simulink model "FOC_Motor_Control"  (R2020b)
settings: Solver=FixedStepDiscrete  StartTime=0.0  StopTime=10.0  FixedStep=Fixed_Step_Size  RelTol=1e-3
values from neighbouring files (symbols this model uses):
  Angle = 1.0    [Hall_HFI_FOC_Data.sldd]
  Cosine_table = 1.0 0.99999529 0.99999058 0.99998587 0.99998116 0.99996704 0.99995291 0.99993885 0.99992472 0.99990118 0.99987763 0.99985409 0.9998306 0.99979764 0.99976468 0.99973178 0.99969882 0.99965644 0.99961412 0.99957174 0.99952942 0.99947762 0.99942589 0.99937415 0.99932235 0.9992612 0.99920005 0.99913889 0.99907768 0.99900717 0.99893659 0.99886602 0.99879545 0.99871546 0.99863547 0.99855554 0.99847555 0.    [Hall_HFI_FOC_Data.sldd]
  Flux = 0.00529276    [Hall_HFI_FOC_Data.sldd]
  HaLL_AngleShift = -0.25    [Hall_HFI_FOC_Data.sldd]
  HaLL_Sector1 = 5.236    [Hall_HFI_FOC_Data.sldd]
  HaLL_Sector2 = 1.0472    [Hall_HFI_FOC_Data.sldd]
  HaLL_Sector3 = 0.0    [Hall_HFI_FOC_Data.sldd]
  HaLL_Sector4 = 3.1415    [Hall_HFI_FOC_Data.sldd]
  HaLL_Sector5 = 4.1888    [Hall_HFI_FOC_Data.sldd]
  HaLL_Sector6 = 2.0944    [Hall_HFI_FOC_Data.sldd]
  HaLL_Timer_T = 1.0E-5    [Hall_HFI_FOC_Data.sldd]
  HFI_bw_BPF = 100.0    [Hall_HFI_FOC_Data.sldd]
  HFI_Fuc_Enalbe = 1.0    [Hall_HFI_FOC_Data.sldd]
  HFI_Inj_HF = 1000.0    [Hall_HFI_FOC_Data.sldd]
  HFI_Inj_HV = 2.0    [Hall_HFI_FOC_Data.sldd]
  HFI_IPD_F = 1000.0    [Hall_HFI_FOC_Data.sldd]
  HFI_IPD_Time = 0.1    [Hall_HFI_FOC_Data.sldd]
  HFI_IPD_V = 1.0    [Hall_HFI_FOC_Data.sldd]
  HFI_NS2RUN_Time = 0.1    [Hall_HFI_FOC_Data.sldd]
  HFI_NS_Low_Time = 0.01    [Hall_HFI_FOC_Data.sldd]
  HFI_NS_Time = 0.05    [Hall_HFI_FOC_Data.sldd]
  HFI_NS_V = 1.0    [Hall_HFI_FOC_Data.sldd]
  HFI_PLL_Omga = 50.0    [Hall_HFI_FOC_Data.sldd]
  HFI_PLL_Xi = 0.707    [Hall_HFI_FOC_Data.sldd]
  HFI_Pulse_Time = 0.001    [Hall_HFI_FOC_Data.sldd]
  HFI_Switch_Time = 0.1    [Hall_HFI_FOC_Data.sldd]
  ID_Ki = 45.0    [Hall_HFI_FOC_Data.sldd]
  ID_Kp = 0.4    [Hall_HFI_FOC_Data.sldd]
  IQ_Ki = 45.0    [Hall_HFI_FOC_Data.sldd]
  IQ_Kp = 0.45    [Hall_HFI_FOC_Data.sldd]
  LADRC_b0 = 80000.0    [Hall_HFI_FOC_Data.sldd]
  LADRC_Omega_c = 80.0    [Hall_HFI_FOC_Data.sldd]
  Ld = 0.0004    [Hall_HFI_FOC_Data.sldd]
  Lq = 0.00045    [Hall_HFI_FOC_Data.sldd]
  Over_modulation = 0.0    [Hall_HFI_FOC_Data.sldd]
  Pole_Pairs = 2.0    [Hall_HFI_FOC_Data.sldd]
  PWM_Frequency = 10000.0    [Hall_HFI_FOC_Data.sldd]
  Sine_table = 0.0 0.0015339879 0.0030679768 0.0046019657 0.0061359555 0.0076698866 0.0092038177 0.010737749 0.012271681 0.013805497 0.015339312 0.016873131 0.018406944 0.019940587 0.021474229 0.023007872 0.024541514 0.026074925 0.027608337 0.029141748 0.03067516 0.032208283 0.033741407 0.035274528 0.036807653 0.038340431 0.039873205 0.04140598 0.042938754 0.04447113 0.046003502 0.047535874 0.049068246 0.0506001    [Hall_HFI_FOC_Data.sldd]
  SMO_PLL_W = 50.0    [Hall_HFI_FOC_Data.sldd]
  Speed_Ki = 0.0633    [Hall_HFI_FOC_Data.sldd]
  Speed_Kp = 0.00867    [Hall_HFI_FOC_Data.sldd]
  Speed_PI_OutputMax = 6.0    [Hall_HFI_FOC_Data.sldd]
  Speed_PI_OutputMin = -6.0    [Hall_HFI_FOC_Data.sldd]
  SpeedFilter_Fn = 0.3    [Hall_HFI_FOC_Data.sldd]
  TorqueMode = 1.0    [Hall_HFI_FOC_Data.sldd]
undefined symbols (not defined in the file or in its folder): DiscIntNeverNeededParam, inverter, magnitude, SVPWM
libraries: simulink x6, eeGeneralControl x3, dspstat3 x3, pid_lib x1
(part 4 of 4)

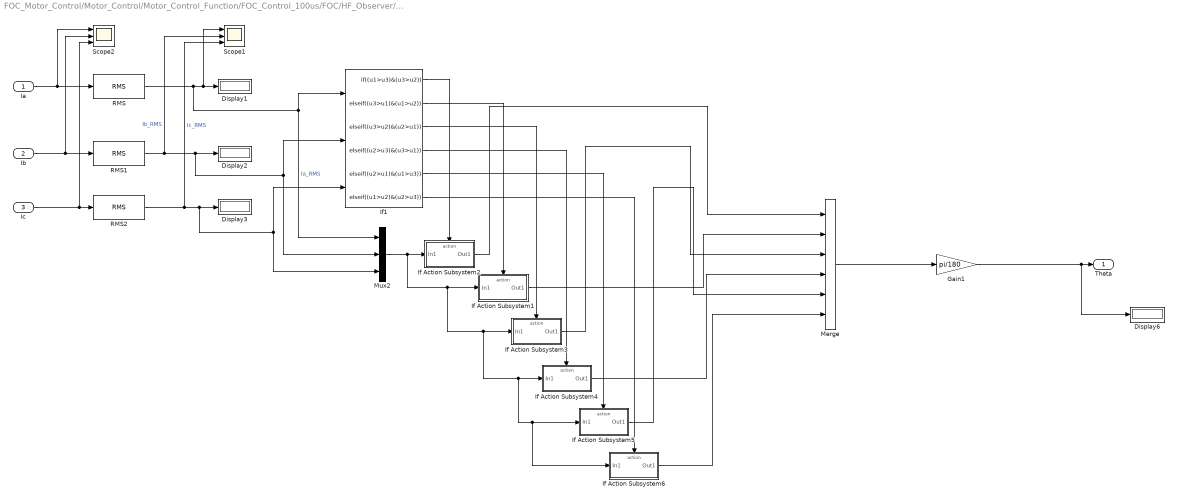
== system FOC_Motor_Control/Motor_Control/Motor_Control_Function/FOC_Control_100us/FOC/HF_Observer/HFI_Function/IPD/Theta_cacl ==
  Ia : Inport
  Ib : Inport  Port=2
  Ic : Inport  Port=3
  Display{1..3,6} (4 alike) : Display
  Gain1 : Gain  Gain=pi/180
  If Action Subsystem1 : Subsystem  TreatAsAtomicUnit=on
  If Action Subsystem2 : Subsystem  TreatAsAtomicUnit=on
  If Action Subsystem3 : Subsystem  TreatAsAtomicUnit=on
  If Action Subsystem4 : Subsystem  TreatAsAtomicUnit=on
  If Action Subsystem5 : Subsystem  TreatAsAtomicUnit=on
  If Action Subsystem6 : Subsystem  TreatAsAtomicUnit=on
  If1 : If  NumInputs=3  IfExpression=(u1>u3)&(u3>u2)  ElseIfExpressions=(u3>u1)&(u1>u2),(u3>u2)&(u2>u1),(u2>u3)&(u3>u1),(u2>u1)&(u1>u3),(u1>u2)&(u2>u3)  ShowElse=off
  Merge : Merge  Inputs=6
  Mux2 : Mux  Inputs=3
  RMS : dspstat3/RMS  run=on  directionMode=Each column  dimension=1  reset_popup=None
  RMS1 : dspstat3/RMS  run=on  directionMode=Each column  dimension=1  reset_popup=None
  RMS2 : dspstat3/RMS  run=on  directionMode=Each column  dimension=1  InputProcessing=Columns as channels (frame based)  reset_popup=None
  Scope1 : Scope  NumInputPorts=3
  Scope2 : Scope  NumInputPorts=3
  Theta : Outport
  wires:
  Ia/1 -> Scope2/1, RMS/1
  Ib/1 -> Scope2/2, RMS1/1
  Ic/1 -> Scope2/3, RMS2/1
  RMS2/1 -> If1/3, Mux2/3, Display3/1, Scope1/3  "Ic_RMS"
  RMS1/1 -> If1/2, Mux2/2, Display2/1, Scope1/2  "Ib_RMS"
  RMS/1 -> If1/1, Mux2/1, Display1/1, Scope1/1  "Ia_RMS"
  If1/1 -> If Action Subsystem2/Action
  If1/2 -> If Action Subsystem1/Action
  If1/3 -> If Action Subsystem3/Action
  If1/4 -> If Action Subsystem4/Action
  If1/5 -> If Action Subsystem5/Action
  If1/6 -> If Action Subsystem6/Action
  Mux2/1 -> If Action Subsystem6/1(In1), If Action Subsystem5/1(In1), If Action Subsystem4/1(In1), If Action Subsystem3/1(In1), If Action Subsystem1/1(In1), If Action Subsystem2/1(In1)
  If Action Subsystem2/1(Out1) -> Merge/1
  If Action Subsystem1/1(Out1) -> Merge/2
  If Action Subsystem3/1(Out1) -> Merge/3
  If Action Subsystem4/1(Out1) -> Merge/4
  If Action Subsystem5/1(Out1) -> Merge/5
  If Action Subsystem6/1(Out1) -> Merge/6
  Merge/1 -> Gain1/1
  Gain1/1 -> Display6/1, Theta/1

== system FOC_Motor_Control/Motor_Control/Motor_Control_Function/FOC_Control_100us/FOC/HF_Observer/HFI_Function/NS/Ud_inject_1 ==
  Theta : Inport
  Action Port : ActionPort  ActionPortLabel=case [ 1 ]:
  1 : Fcn  Expr=u[1]*u[4]-u[2]*u[3]
  2 : Fcn  Expr=u[1]*u[3]+u[2]*u[4]
  Constant : Constant  Value=0  OutDataTypeStr=single
  Constant2 : Constant  Value=0  OutDataTypeStr=single
  Mux : Mux
  Sine_Cosine : Subsystem  TreatAsAtomicUnit=on
      settings: RTWSystemCode=Nonreusable function  RTWFcnNameOpts=Use subsystem name
  Ualpha : Outport
  Ubeta : Outport  Port=2
  wires:
  Constant2/1 -> Mux/2
  Theta/1 -> Sine_Cosine/1(P)
  2/1 -> Ubeta/1
  Sine_Cosine/2(Cos) -> Mux/4
  1/1 -> Ualpha/1
  Constant/1 -> Mux/1
  Mux/1 -> 2/1, 1/1
  Sine_Cosine/1(Sin) -> Mux/3

== system FOC_Motor_Control/Motor_Control/Motor_Control_Function/FOC_Control_100us/FOC/HF_Observer/HFI_Function/NS/Ud_inject_2 ==
  Id : Inport
  Theta : Inport  Port=2
  Action Port : ActionPort  ActionPortLabel=case [ 2 ]:
  1 : Fcn  Expr=u[1]*u[4]-u[2]*u[3]
  2 : Fcn  Expr=u[1]*u[3]+u[2]*u[4]
  Constant : Constant  Value=HFI_NS_V  OutDataTypeStr=single
  Constant2 : Constant  Value=0  OutDataTypeStr=single
  Mux : Mux
  Sine_Cosine : Subsystem  TreatAsAtomicUnit=on
      settings: RTWSystemCode=Nonreusable function  RTWFcnNameOpts=Use subsystem name
  Ualpha : Outport
  Ubeta : Outport  Port=2
  Id_out : Outport  Port=3
  wires:
  Constant2/1 -> Mux/2
  Theta/1 -> Sine_Cosine/1(P)
  2/1 -> Ubeta/1
  Sine_Cosine/2(Cos) -> Mux/4
  1/1 -> Ualpha/1
  Constant/1 -> Mux/1
  Mux/1 -> 2/1, 1/1
  Sine_Cosine/1(Sin) -> Mux/3
  Id/1 -> Id_out/1

== system FOC_Motor_Control/Motor_Control/Motor_Control_Function/FOC_Control_100us/FOC/HF_Observer/HFI_Function/NS/Ud_inject_3 ==
  Theta : Inport
  Action Port : ActionPort  ActionPortLabel=case [ 3 ]:
  1 : Fcn  Expr=u[1]*u[4]-u[2]*u[3]
  2 : Fcn  Expr=u[1]*u[3]+u[2]*u[4]
  Constant : Constant  Value=0  OutDataTypeStr=single
  Constant2 : Constant  Value=0  OutDataTypeStr=single
  Mux : Mux
  Sine_Cosine : Subsystem  TreatAsAtomicUnit=on
      settings: RTWSystemCode=Nonreusable function  RTWFcnNameOpts=Use subsystem name
  Ualpha : Outport
  Ubeta : Outport  Port=2
  wires:
  Constant2/1 -> Mux/2
  Theta/1 -> Sine_Cosine/1(P)
  2/1 -> Ubeta/1
  Sine_Cosine/2(Cos) -> Mux/4
  1/1 -> Ualpha/1
  Constant/1 -> Mux/1
  Mux/1 -> 2/1, 1/1
  Sine_Cosine/1(Sin) -> Mux/3

== system FOC_Motor_Control/Motor_Control/Motor_Control_Function/FOC_Control_100us/FOC/HF_Observer/HFI_Function/NS/Ud_inject_4 ==
  Id : Inport
  Theta : Inport  Port=2
  Action Port : ActionPort  ActionPortLabel=case [ 4 ]:
  1 : Fcn  Expr=u[1]*u[4]-u[2]*u[3]
  2 : Fcn  Expr=u[1]*u[3]+u[2]*u[4]
  Constant : Constant  Value=HFI_NS_V  OutDataTypeStr=single
  Constant2 : Constant  Value=0  OutDataTypeStr=single
  Mux : Mux
  Sine_Cosine : Subsystem  TreatAsAtomicUnit=on
      settings: RTWSystemCode=Nonreusable function
  Theta_limit : Subsystem
      settings: RTWSystemCode=Nonreusable function
  Ualpha : Outport
  Ubeta : Outport  Port=2
  Id_out : Outport  Port=3
  wires:
  Constant2/1 -> Mux/2
  2/1 -> Ubeta/1
  Sine_Cosine/2(Cos) -> Mux/4
  1/1 -> Ualpha/1
  Constant/1 -> Mux/1
  Mux/1 -> 2/1, 1/1
  Sine_Cosine/1(Sin) -> Mux/3
  Id/1 -> Id_out/1
  Theta_limit/1(Angle_output) -> Sine_Cosine/1(P)
  Theta/1 -> Theta_limit/1(Angle_input)

== system FOC_Motor_Control/Motor_Control/Motor_Control_Function/FOC_Control_100us/FOC/HF_Observer/HFI_Function/NS/Ud_inject_5 ==
  Theta : Inport
  Id1 : Inport  Port=2
  Id2 : Inport  Port=3
  Action Port : ActionPort  ActionPortLabel=case [ 5 ]:
  1 : Fcn  Expr=u[1]*u[4]-u[2]*u[3]
  2 : Fcn  Expr=u[1]*u[3]+u[2]*u[4]
  Constant : Constant  Value=0  OutDataTypeStr=single
  Constant2 : Constant  Value=0  OutDataTypeStr=single
  If1 : If  NumInputs=2  IfExpression=u1>=u2  ElseIfExpressions=u1<u2  ShowElse=off
  Merge1 : Merge
  Mux : Mux
  Sine_Cosine : Subsystem
      settings: RTWSystemCode=Nonreusable function  RTWFcnNameOpts=Use subsystem name
  Subsystem : Subsystem
  Subsystem1 : Subsystem
  Ualpha : Outport
  Ubeta : Outport  Port=2
  IPD_Angle : Outport  Port=3
  wires:
  Constant2/1 -> Mux/2
  Theta/1 -> Subsystem1/1(In1), Subsystem/1(In1), Sine_Cosine/1(P)
  2/1 -> Ubeta/1
  Sine_Cosine/2(Cos) -> Mux/4
  1/1 -> Ualpha/1
  Constant/1 -> Mux/1
  Mux/1 -> 2/1, 1/1
  Sine_Cosine/1(Sin) -> Mux/3
  Id1/1 -> If1/1
  Id2/1 -> If1/2
  If1/1 -> Subsystem/Action
  If1/2 -> Subsystem1/Action
  Subsystem/1(Out1) -> Merge1/1
  Subsystem1/1(Out1) -> Merge1/2
  Merge1/1 -> IPD_Angle/1

== system FOC_Motor_Control/Motor_Control/Motor_Control_Function/FOC_Control_100us/FOC/HF_Observer/HFI_Function/HFI/IPD_Angle/Angle_calibration ==
  Angle_input : Inport
  Angle_offset : Constant  Value=-pi  OutDataTypeStr=single
  If Action Subsystem1 : Subsystem  TreatAsAtomicUnit=on
  If Action Subsystem2 : Subsystem  TreatAsAtomicUnit=on
  If Action Subsystem3 : Subsystem  TreatAsAtomicUnit=on
  If1 : If  IfExpression=u1 > 6.283185307  ElseIfExpressions=u1<0
  Merge1 : Merge  Inputs=3
  Subtract1 : Sum
  Angle_output : Outport
  wires:
  Angle_input/1 -> Subtract1/1
  Angle_offset/1 -> Subtract1/2  "Control_ModeCommand"
  If1/1 -> If Action Subsystem2/Action
  If1/3 -> If Action Subsystem1/Action
  If Action Subsystem2/1(Out1) -> Merge1/1
  Subtract1/1 -> If Action Subsystem3/1(In1), If Action Subsystem1/1(In1), If Action Subsystem2/1(In1), If1/1
  If Action Subsystem1/1(Out1) -> Merge1/3
  If Action Subsystem3/1(Out1) -> Merge1/2
  If1/2 -> If Action Subsystem3/Action
  Merge1/1 -> Angle_output/1

== system FOC_Motor_Control/Motor_Control/Motor_Control_Function/FOC_Control_100us/FOC/HF_Observer/HFI_Function/HFI/IPD_Angle1/Angle_calibration ==
  Angle_input : Inport
  Angle_offset : Constant  Value=pi  OutDataTypeStr=single
  If Action Subsystem1 : Subsystem  TreatAsAtomicUnit=on
  If Action Subsystem2 : Subsystem  TreatAsAtomicUnit=on
  If Action Subsystem3 : Subsystem  TreatAsAtomicUnit=on
  If1 : If  IfExpression=u1 > 6.283185307  ElseIfExpressions=u1<0
  Merge1 : Merge  Inputs=3
  Subtract1 : Sum
  Angle_output : Outport
  wires:
  Angle_input/1 -> Subtract1/1
  Angle_offset/1 -> Subtract1/2  "Control_ModeCommand"
  If1/1 -> If Action Subsystem2/Action
  If1/3 -> If Action Subsystem1/Action
  If Action Subsystem2/1(Out1) -> Merge1/1
  Subtract1/1 -> If Action Subsystem3/1(In1), If Action Subsystem1/1(In1), If Action Subsystem2/1(In1), If1/1
  If Action Subsystem1/1(Out1) -> Merge1/3
  If Action Subsystem3/1(Out1) -> Merge1/2
  If1/2 -> If Action Subsystem3/Action
  Merge1/1 -> Angle_output/1

== system FOC_Motor_Control/Motor_Control/Motor_Control_Function/FOC_Control_100us/FOC/HF_Observer/HFI_Function/HFI/Subsystem/Sine_Cosine ==
  note: Sine Cosine Coefficients
  P : Inport
  Cosine : Lookup_n-D  NumberOfTableDimensions=1  LookupTableObject=''  BreakpointsForDimension1=[0:2*pi/4095:2*pi]  BreakpointsForDimension1FirstPoint=10  BreakpointsForDimension2FirstPoint=10  BreakpointsForDimension1Spacing=12  BreakpointsForDimension2Spacing=12  IndexSearchMethod=Evenly spaced points  Table=Cosine_table  InterpMethod=Flat  DiagnosticForOutOfRangeInput=Error  InternalRulePriority=Speed  RndMeth=Simplest  InputSameDT=on
  Saturation : Saturate  UpperLimit=2*pi-0.001  LowerLimit=0+0.001
  Scope : Scope  NumInputPorts=2
  Sine : Lookup_n-D  NumberOfTableDimensions=1  LookupTableObject=''  BreakpointsForDimension1=[0:2*pi/4095:2*pi]  BreakpointsForDimension1FirstPoint=10  BreakpointsForDimension2FirstPoint=10  BreakpointsForDimension1Spacing=12  BreakpointsForDimension2Spacing=12  IndexSearchMethod=Evenly spaced points  Table=Sine_table  InterpMethod=Flat  DiagnosticForOutOfRangeInput=Error  InternalRulePriority=Speed  RndMeth=Simplest  InputSameDT=on
  Sin : Outport  VectorParamsAs1DForOutWhenUnconnected=off
  Cos : Outport  Port=2  VectorParamsAs1DForOutWhenUnconnected=off
  wires:
  P/1 -> Saturation/1  "position"
  Sine/1 -> Scope/1, Sin/1
  Cosine/1 -> Scope/2, Cos/1
  Saturation/1 -> Cosine/1, Sine/1

== system FOC_Motor_Control/Motor_Control/Motor_Control_Function/FOC_Control_100us/FOC/HF_Observer/HFI_Function/IPD/Theta_cacl/If Action Subsystem1 ==
  In1 : Inport
  Action Port : ActionPort  ActionPortLabel=elseif((u3>u1)&(u1>u2))
  Fcn : Fcn  Expr=(u(3)-u(1))/(u(3)-u(2))*30+30
  Out1 : Outport
  wires:
  In1/1 -> Fcn/1
  Fcn/1 -> Out1/1

== system FOC_Motor_Control/Motor_Control/Motor_Control_Function/FOC_Control_100us/FOC/HF_Observer/HFI_Function/IPD/Theta_cacl/If Action Subsystem2 ==
  In1 : Inport
  Action Port : ActionPort  ActionPortLabel=if((u1>u3)&(u3>u2))
  Fcn : Fcn  Expr=(u(3)-u(2))/(u(1)-u(2))*30
  Out1 : Outport
  wires:
  In1/1 -> Fcn/1
  Fcn/1 -> Out1/1

== system FOC_Motor_Control/Motor_Control/Motor_Control_Function/FOC_Control_100us/FOC/HF_Observer/HFI_Function/IPD/Theta_cacl/If Action Subsystem3 ==
  In1 : Inport
  Action Port : ActionPort  ActionPortLabel=elseif((u3>u2)&(u2>u1))
  Fcn : Fcn  Expr=(u(2)-u(1))/(u(3)-u(1))*30+60
  Out1 : Outport
  wires:
  In1/1 -> Fcn/1
  Fcn/1 -> Out1/1

== system FOC_Motor_Control/Motor_Control/Motor_Control_Function/FOC_Control_100us/FOC/HF_Observer/HFI_Function/IPD/Theta_cacl/If Action Subsystem4 ==
  In1 : Inport
  Action Port : ActionPort  ActionPortLabel=elseif((u2>u3)&(u3>u1))
  Fcn : Fcn  Expr=(u(2)-u(3))/(u(2)-u(1))*30+90
  Out1 : Outport
  wires:
  In1/1 -> Fcn/1
  Fcn/1 -> Out1/1

== system FOC_Motor_Control/Motor_Control/Motor_Control_Function/FOC_Control_100us/FOC/HF_Observer/HFI_Function/IPD/Theta_cacl/If Action Subsystem5 ==
  In1 : Inport
  Action Port : ActionPort  ActionPortLabel=elseif((u2>u1)&(u1>u3))
  Fcn : Fcn  Expr=(u(1)-u(3))/(u(2)-u(3))*30+120
  Out1 : Outport
  wires:
  In1/1 -> Fcn/1
  Fcn/1 -> Out1/1

== system FOC_Motor_Control/Motor_Control/Motor_Control_Function/FOC_Control_100us/FOC/HF_Observer/HFI_Function/IPD/Theta_cacl/If Action Subsystem6 ==
  In1 : Inport
  Action Port : ActionPort  ActionPortLabel=elseif((u1>u2)&(u2>u3))
  Fcn : Fcn  Expr=(u(1)-u(2))/(u(1)-u(3))*30+150
  Out1 : Outport
  wires:
  In1/1 -> Fcn/1
  Fcn/1 -> Out1/1

== system FOC_Motor_Control/Motor_Control/Motor_Control_Function/FOC_Control_100us/FOC/HF_Observer/HFI_Function/NS/Ud_inject_1/Sine_Cosine ==
  note: Sine Cosine Coefficients
  P : Inport
  Cosine : Lookup_n-D  NumberOfTableDimensions=1  LookupTableObject=''  BreakpointsForDimension1=[0:2*pi/4095:2*pi]  BreakpointsForDimension1FirstPoint=10  BreakpointsForDimension2FirstPoint=10  BreakpointsForDimension1Spacing=12  BreakpointsForDimension2Spacing=12  IndexSearchMethod=Evenly spaced points  Table=Cosine_table  InterpMethod=Flat  DiagnosticForOutOfRangeInput=Error  InternalRulePriority=Speed  RndMeth=Simplest  InputSameDT=on
  Scope : Scope  NumInputPorts=2
  Sine : Lookup_n-D  NumberOfTableDimensions=1  LookupTableObject=''  BreakpointsForDimension1=[0:2*pi/4095:2*pi]  BreakpointsForDimension1FirstPoint=10  BreakpointsForDimension2FirstPoint=10  BreakpointsForDimension1Spacing=12  BreakpointsForDimension2Spacing=12  IndexSearchMethod=Evenly spaced points  Table=Sine_table  InterpMethod=Flat  DiagnosticForOutOfRangeInput=Error  InternalRulePriority=Speed  RndMeth=Simplest  InputSameDT=on
  Sin : Outport  VectorParamsAs1DForOutWhenUnconnected=off
  Cos : Outport  Port=2  VectorParamsAs1DForOutWhenUnconnected=off
  wires:
  P/1 -> Cosine/1, Sine/1  "position"
  Sine/1 -> Scope/1, Sin/1
  Cosine/1 -> Scope/2, Cos/1

== system FOC_Motor_Control/Motor_Control/Motor_Control_Function/FOC_Control_100us/FOC/HF_Observer/HFI_Function/NS/Ud_inject_2/Sine_Cosine ==
  note: Sine Cosine Coefficients
  P : Inport
  Cosine : Lookup_n-D  NumberOfTableDimensions=1  LookupTableObject=''  BreakpointsForDimension1=[0:2*pi/4095:2*pi]  BreakpointsForDimension1FirstPoint=10  BreakpointsForDimension2FirstPoint=10  BreakpointsForDimension1Spacing=12  BreakpointsForDimension2Spacing=12  IndexSearchMethod=Evenly spaced points  Table=Cosine_table  InterpMethod=Flat  DiagnosticForOutOfRangeInput=Error  InternalRulePriority=Speed  RndMeth=Simplest  InputSameDT=on
  Scope : Scope  NumInputPorts=2
  Sine : Lookup_n-D  NumberOfTableDimensions=1  LookupTableObject=''  BreakpointsForDimension1=[0:2*pi/4095:2*pi]  BreakpointsForDimension1FirstPoint=10  BreakpointsForDimension2FirstPoint=10  BreakpointsForDimension1Spacing=12  BreakpointsForDimension2Spacing=12  IndexSearchMethod=Evenly spaced points  Table=Sine_table  InterpMethod=Flat  DiagnosticForOutOfRangeInput=Error  InternalRulePriority=Speed  RndMeth=Simplest  InputSameDT=on
  Sin : Outport  VectorParamsAs1DForOutWhenUnconnected=off
  Cos : Outport  Port=2  VectorParamsAs1DForOutWhenUnconnected=off
  wires:
  P/1 -> Cosine/1, Sine/1  "position"
  Sine/1 -> Scope/1, Sin/1
  Cosine/1 -> Scope/2, Cos/1

== system FOC_Motor_Control/Motor_Control/Motor_Control_Function/FOC_Control_100us/FOC/HF_Observer/HFI_Function/NS/Ud_inject_3/Sine_Cosine ==
  note: Sine Cosine Coefficients
  P : Inport
  Cosine : Lookup_n-D  NumberOfTableDimensions=1  LookupTableObject=''  BreakpointsForDimension1=[0:2*pi/4095:2*pi]  BreakpointsForDimension1FirstPoint=10  BreakpointsForDimension2FirstPoint=10  BreakpointsForDimension1Spacing=12  BreakpointsForDimension2Spacing=12  IndexSearchMethod=Evenly spaced points  Table=Cosine_table  InterpMethod=Flat  DiagnosticForOutOfRangeInput=Error  InternalRulePriority=Speed  RndMeth=Simplest  InputSameDT=on
  Scope : Scope  NumInputPorts=2
  Sine : Lookup_n-D  NumberOfTableDimensions=1  LookupTableObject=''  BreakpointsForDimension1=[0:2*pi/4095:2*pi]  BreakpointsForDimension1FirstPoint=10  BreakpointsForDimension2FirstPoint=10  BreakpointsForDimension1Spacing=12  BreakpointsForDimension2Spacing=12  IndexSearchMethod=Evenly spaced points  Table=Sine_table  InterpMethod=Flat  DiagnosticForOutOfRangeInput=Error  InternalRulePriority=Speed  RndMeth=Simplest  InputSameDT=on
  Sin : Outport  VectorParamsAs1DForOutWhenUnconnected=off
  Cos : Outport  Port=2  VectorParamsAs1DForOutWhenUnconnected=off
  wires:
  P/1 -> Cosine/1, Sine/1  "position"
  Sine/1 -> Scope/1, Sin/1
  Cosine/1 -> Scope/2, Cos/1

== system FOC_Motor_Control/Motor_Control/Motor_Control_Function/FOC_Control_100us/FOC/HF_Observer/HFI_Function/NS/Ud_inject_4/Sine_Cosine ==
  note: Sine Cosine Coefficients
  P : Inport
  Cosine : Lookup_n-D  NumberOfTableDimensions=1  LookupTableObject=''  BreakpointsForDimension1=[0:2*pi/4095:2*pi]  BreakpointsForDimension1FirstPoint=10  BreakpointsForDimension2FirstPoint=10  BreakpointsForDimension1Spacing=12  BreakpointsForDimension2Spacing=12  IndexSearchMethod=Evenly spaced points  Table=Cosine_table  InterpMethod=Flat  DiagnosticForOutOfRangeInput=Error  InternalRulePriority=Speed  RndMeth=Simplest  InputSameDT=on
  Scope : Scope  NumInputPorts=2
  Sine : Lookup_n-D  NumberOfTableDimensions=1  LookupTableObject=''  BreakpointsForDimension1=[0:2*pi/4095:2*pi]  BreakpointsForDimension1FirstPoint=10  BreakpointsForDimension2FirstPoint=10  BreakpointsForDimension1Spacing=12  BreakpointsForDimension2Spacing=12  IndexSearchMethod=Evenly spaced points  Table=Sine_table  InterpMethod=Flat  DiagnosticForOutOfRangeInput=Error  InternalRulePriority=Speed  RndMeth=Simplest  InputSameDT=on
  Sin : Outport  VectorParamsAs1DForOutWhenUnconnected=off
  Cos : Outport  Port=2  VectorParamsAs1DForOutWhenUnconnected=off
  wires:
  P/1 -> Cosine/1, Sine/1  "position"
  Sine/1 -> Scope/1, Sin/1
  Cosine/1 -> Scope/2, Cos/1

== system FOC_Motor_Control/Motor_Control/Motor_Control_Function/FOC_Control_100us/FOC/HF_Observer/HFI_Function/NS/Ud_inject_4/Theta_limit ==
  Angle_input : Inport
  Angle_offset : Constant  Value=pi  OutDataTypeStr=single
  If Action Subsystem1 : Subsystem  TreatAsAtomicUnit=on
  If Action Subsystem2 : Subsystem  TreatAsAtomicUnit=on
  If1 : If  IfExpression=u1 > 6.283185307
  Merge1 : Merge
  Subtract1 : Sum
  Angle_output : Outport
  wires:
  Angle_input/1 -> Subtract1/1
  Merge1/1 -> Angle_output/1
  Angle_offset/1 -> Subtract1/2
  If1/1 -> If Action Subsystem2/Action
  If1/2 -> If Action Subsystem1/Action
  If Action Subsystem2/1(Out1) -> Merge1/1
  Subtract1/1 -> If Action Subsystem1/1(In1), If Action Subsystem2/1(In1), If1/1
  If Action Subsystem1/1(Out1) -> Merge1/2

== system FOC_Motor_Control/Motor_Control/Motor_Control_Function/FOC_Control_100us/FOC/HF_Observer/HFI_Function/NS/Ud_inject_5/Sine_Cosine ==
  note: Sine Cosine Coefficients
  P : Inport
  Cosine : Lookup_n-D  NumberOfTableDimensions=1  LookupTableObject=''  BreakpointsForDimension1=[0:2*pi/4095:2*pi]  BreakpointsForDimension1FirstPoint=10  BreakpointsForDimension2FirstPoint=10  BreakpointsForDimension1Spacing=12  BreakpointsForDimension2Spacing=12  IndexSearchMethod=Evenly spaced points  Table=Cosine_table  InterpMethod=Flat  DiagnosticForOutOfRangeInput=Error  InternalRulePriority=Speed  RndMeth=Simplest  InputSameDT=on
  Scope : Scope  NumInputPorts=2
  Sine : Lookup_n-D  NumberOfTableDimensions=1  LookupTableObject=''  BreakpointsForDimension1=[0:2*pi/4095:2*pi]  BreakpointsForDimension1FirstPoint=10  BreakpointsForDimension2FirstPoint=10  BreakpointsForDimension1Spacing=12  BreakpointsForDimension2Spacing=12  IndexSearchMethod=Evenly spaced points  Table=Sine_table  InterpMethod=Flat  DiagnosticForOutOfRangeInput=Error  InternalRulePriority=Speed  RndMeth=Simplest  InputSameDT=on
  Sin : Outport  VectorParamsAs1DForOutWhenUnconnected=off
  Cos : Outport  Port=2  VectorParamsAs1DForOutWhenUnconnected=off
  wires:
  P/1 -> Cosine/1, Sine/1  "position"
  Sine/1 -> Scope/1, Sin/1
  Cosine/1 -> Scope/2, Cos/1

== system FOC_Motor_Control/Motor_Control/Motor_Control_Function/FOC_Control_100us/FOC/HF_Observer/HFI_Function/NS/Ud_inject_5/Subsystem ==
  In1 : Inport
  Action Port : ActionPort  ActionPortLabel=if(u1>=u2)
  Out1 : Outport
  wires:
  In1/1 -> Out1/1

== system FOC_Motor_Control/Motor_Control/Motor_Control_Function/FOC_Control_100us/FOC/HF_Observer/HFI_Function/NS/Ud_inject_5/Subsystem1 ==
  In1 : Inport
  Action Port : ActionPort  ActionPortLabel=elseif(u1<u2)
  Theta_limit : Subsystem
      settings: RTWSystemCode=Nonreusable function  RTWFcnNameOpts=Use subsystem name
  Out1 : Outport
  wires:
  In1/1 -> Theta_limit/1(Angle_input)
  Theta_limit/1(Angle_output) -> Out1/1

== system FOC_Motor_Control/Motor_Control/Motor_Control_Function/FOC_Control_100us/FOC/HF_Observer/HFI_Function/HFI/IPD_Angle/Angle_calibration/If Action Subsystem1 ==
  In1 : Inport
  Action Port : ActionPort  ActionPortLabel=else
  Out1 : Outport
  wires:
  In1/1 -> Out1/1

== system FOC_Motor_Control/Motor_Control/Motor_Control_Function/FOC_Control_100us/FOC/HF_Observer/HFI_Function/HFI/IPD_Angle/Angle_calibration/If Action Subsystem2 ==
  In1 : Inport
  Action Port : ActionPort  ActionPortLabel=if(u1 > 6.283185307)
  2pi : Constant  Value=2*pi  OutDataTypeStr=single
  Subtract1 : Sum  Inputs=+-  OutDataTypeStr=single
  Out1 : Outport
  wires:
  In1/1 -> Subtract1/1
  Subtract1/1 -> Out1/1
  2pi/1 -> Subtract1/2

== system FOC_Motor_Control/Motor_Control/Motor_Control_Function/FOC_Control_100us/FOC/HF_Observer/HFI_Function/HFI/IPD_Angle/Angle_calibration/If Action Subsystem3 ==
  In1 : Inport
  Action Port : ActionPort  ActionPortLabel=elseif(u1<0)
  Angle_offset : Constant  Value=2*pi  OutDataTypeStr=single
  Subtract1 : Sum
  Out1 : Outport
  wires:
  In1/1 -> Subtract1/1
  Subtract1/1 -> Out1/1
  Angle_offset/1 -> Subtract1/2

== system FOC_Motor_Control/Motor_Control/Motor_Control_Function/FOC_Control_100us/FOC/HF_Observer/HFI_Function/HFI/IPD_Angle1/Angle_calibration/If Action Subsystem1 ==
  In1 : Inport
  Action Port : ActionPort  ActionPortLabel=else
  Out1 : Outport
  wires:
  In1/1 -> Out1/1

== system FOC_Motor_Control/Motor_Control/Motor_Control_Function/FOC_Control_100us/FOC/HF_Observer/HFI_Function/HFI/IPD_Angle1/Angle_calibration/If Action Subsystem2 ==
  In1 : Inport
  Action Port : ActionPort  ActionPortLabel=if(u1 > 6.283185307)
  2pi : Constant  Value=2*pi  OutDataTypeStr=single
  Subtract1 : Sum  Inputs=+-  OutDataTypeStr=single
  Out1 : Outport
  wires:
  In1/1 -> Subtract1/1
  Subtract1/1 -> Out1/1
  2pi/1 -> Subtract1/2

== system FOC_Motor_Control/Motor_Control/Motor_Control_Function/FOC_Control_100us/FOC/HF_Observer/HFI_Function/HFI/IPD_Angle1/Angle_calibration/If Action Subsystem3 ==
  In1 : Inport
  Action Port : ActionPort  ActionPortLabel=elseif(u1<0)
  Angle_offset : Constant  Value=2*pi  OutDataTypeStr=single
  Subtract1 : Sum
  Out1 : Outport
  wires:
  In1/1 -> Subtract1/1
  Subtract1/1 -> Out1/1
  Angle_offset/1 -> Subtract1/2

== system FOC_Motor_Control/Motor_Control/Motor_Control_Function/FOC_Control_100us/FOC/HF_Observer/HFI_Function/NS/Ud_inject_4/Theta_limit/If Action Subsystem1 ==
  In1 : Inport
  Action Port : ActionPort  ActionPortLabel=else
  Out1 : Outport
  wires:
  In1/1 -> Out1/1

== system FOC_Motor_Control/Motor_Control/Motor_Control_Function/FOC_Control_100us/FOC/HF_Observer/HFI_Function/NS/Ud_inject_4/Theta_limit/If Action Subsystem2 ==
  In1 : Inport
  Action Port : ActionPort  ActionPortLabel=if(u1 > 6.283185307)
  2pi : Constant  Value=2*pi  OutDataTypeStr=single
  Subtract1 : Sum  Inputs=+-
  Out1 : Outport
  wires:
  In1/1 -> Subtract1/1
  Subtract1/1 -> Out1/1
  2pi/1 -> Subtract1/2

== system FOC_Motor_Control/Motor_Control/Motor_Control_Function/FOC_Control_100us/FOC/HF_Observer/HFI_Function/NS/Ud_inject_5/Subsystem1/Theta_limit ==
  Angle_input : Inport
  Angle_offset : Constant  Value=pi  OutDataTypeStr=single
  If Action Subsystem1 : Subsystem  TreatAsAtomicUnit=on
  If Action Subsystem2 : Subsystem  TreatAsAtomicUnit=on
  If1 : If  IfExpression=u1 > 6.283185307
  Merge1 : Merge
  Subtract1 : Sum
  Angle_output : Outport
  wires:
  Angle_input/1 -> Subtract1/1
  Merge1/1 -> Angle_output/1
  Angle_offset/1 -> Subtract1/2
  If1/1 -> If Action Subsystem2/Action
  If1/2 -> If Action Subsystem1/Action
  If Action Subsystem2/1(Out1) -> Merge1/1
  Subtract1/1 -> If Action Subsystem1/1(In1), If Action Subsystem2/1(In1), If1/1
  If Action Subsystem1/1(Out1) -> Merge1/2

== system FOC_Motor_Control/Motor_Control/Motor_Control_Function/FOC_Control_100us/FOC/HF_Observer/HFI_Function/NS/Ud_inject_5/Subsystem1/Theta_limit/If Action Subsystem1 ==
  In1 : Inport
  Action Port : ActionPort  ActionPortLabel=else
  Out1 : Outport
  wires:
  In1/1 -> Out1/1

== system FOC_Motor_Control/Motor_Control/Motor_Control_Function/FOC_Control_100us/FOC/HF_Observer/HFI_Function/NS/Ud_inject_5/Subsystem1/Theta_limit/If Action Subsystem2 ==
  In1 : Inport
  Action Port : ActionPort  ActionPortLabel=if(u1 > 6.283185307)
  2pi : Constant  Value=2*pi  OutDataTypeStr=single
  Subtract1 : Sum  Inputs=+-
  Out1 : Outport
  wires:
  In1/1 -> Subtract1/1
  Subtract1/1 -> Out1/1
  2pi/1 -> Subtract1/2

== stateflow chart FOC_Motor_Control/Motor_Control/Motor_Control_Function/FOC_Control_100us/FOC/HF_Observer/HFI_Function/HFI_State_machine ==
  note: [HFI_flag==1]
  state HFI_NS
    en: HFI_state=2;
    NS_flag=1;
  state HFI_IPD
    en: HFI_state = 1;
    IPD_flag=1;
  state HFI_RUN
    en:HFI_state=3;
    HFI_RUN_flag=1;
  (default) -> HFI_IPD
  HFI_IPD -> HFI_NS : [after(HFI_IPD_Time,sec) &HFI_flag==1 & IPD_flag==1]
  HFI_NS -> HFI_RUN : [after(HFI_NS_Time,sec) & NS_flag==1]
  data: HFI_flag input; HFI_state output uint8; IPD_flag local; NS_flag local; HFI_RUN_flag local; NS_RUN_flag local; HFI_IPD_Time input; HFI_NS_Time input

== stateflow chart FOC_Motor_Control/Motor_Control/Motor_Control_Function/FOC_Control_100us/FOC/HF_Observer/HFI_Function/NS/NS_State_machine ==
  note: NS_flag==1]
  state NS_2
    en: NS_state=2;
    NS_2_flag=1;
  state NS_1
    en: NS_state = 1;
    NS_1_flag=1;
  state NS_3
    en: NS_state=3;
    NS_3_flag=1;
  state NS_4
    en: NS_state=4;
    NS_4_flag=1;
  state NS_5
    en: NS_state=5;
    NS_5_flag=1;
  (default) -> NS_1
  NS_1 -> NS_2 : [after(HFI_NS_Low_Time,sec) &NS_1_flag==1 ]
  NS_2 -> NS_3 : [after(HFI_NS_Pulse_Time,sec) &NS_2_flag==1 ]
  NS_3 -> NS_4 : [after(HFI_NS_Low_Time,sec) &NS_3_flag==1]
  NS_4 -> NS_5 : [after(HFI_NS_Pulse_Time,sec) &NS_4_flag==1]
  data: NS_flag1 input; NS_state output uint8; NS_1_flag local; NS_2_flag local; NS_3_flag local; NS_4_flag local; NS_5_flag local; HFI_NS_Low_Time input; HFI_NS_Pulse_Time input

== stateflow chart FOC_Motor_Control/Motor_Control/Motor_Control_Function/FOC_Control_100us/FOC/HF_Observer/HFI_Function/HFI/StartRUN_State_machine ==
  note: [RUN_flag==1]
  state NS_2_RUN
    en: RUN_state = 1;
    NS_RUN_flag=1;
  state Start_RUN
    en: RUN_state=2;
    Switch_flag=1;
  state RUN
    en: RUN_state=3;
    Start_RUN_flag=1;
  (default) -> NS_2_RUN
  NS_2_RUN -> Start_RUN : [after(HFI_NS2RUN_Time,sec) &NS_RUN_flag==1]
  Start_RUN -> RUN : [after(HFI_Switch_Time,sec) &Switch_flag==1]
  data: RUN_state output uint8; NS_RUN_flag local; Start_RUN_flag local; RUN_flag input; Switch_flag local; HFI_Switch_Time input; HFI_NS2RUN_Time input
